simulink model "enginespeed_qat_mlfcn"  (R2025b)
settings: Solver=ode23  StartTime=0.0  StopTime=25  FixedStep=0.1  MaxStep=0.01  RelTol=1e-3  EnableMultiTasking=on
model workspace (MAT data in the model file):
  p = [-7.82997288351e-05; 0.181210895977; -0.072497134344; 0.000486358314052; 0.0361674637937]
settings Model: Creator=The MathWorks, Inc.  LastModifiedBy=arkadiyturevskiy
settings SolverCC: ZeroCrossAlgorithm=Non-adaptive  AlgebraicLoopSolver=TrustRegion
settings DataIOCC: LimitDataPoints=on  SaveFormat=Array  SaveOutput=off  SaveTime=off  ReturnWorkspaceOutputs=off
settings OptimizationCC: DefaultParameterBehavior=Inlined  InlineInvariantSignals=on  BufferReuse=off  ReuseModelBlockBuffer=off  ExpressionDepthLimit=2147483647.0  InitFltsAndDblsToZero=on  EfficientMapNaN2IntZero=off  LifeSpan=inf
settings DebuggingCC: SaveWithParameterizedLinksMsg=none  UnderspecifiedInitializationDetection=Classic  MergeDetectMultiDrivingBlocksExec=none  CheckExecutionContextPreStartOutputMsg=on  SignalResolutionControl=TryResolveAllWithWarning  MultiTaskDSMMsg=warning  FcnCallInpInsideContextMsg=warning  UnconnectedInputMsg=warning  UnconnectedOutputMsg=warning  UnconnectedLineMsg=warning  StateNameClashWarn=warning  SubsystemReferenceDiagnosticForUnitTest=warning  SFUnexpectedBacktrackingDiag=warning  SFNoUnconditionalDefaultTransitionDiag=warning  SFExecutionAtInitializationDiag=none  ArithmeticOperatorsInVariantConditions=warning
settings HardwareCC: ProdBitPerPointer=32.0  ProdBitPerSizeT=32.0  ProdBitPerPtrDiffT=32.0  ProdLargestAtomicFloat=None  ProdIntDivRoundTo=Undefined  ProdEndianess=Unspecified  ProdWordSize=32.0  ProdHWDeviceType=32-bit Generic
settings ModelReferenceCC: PropagateSignalLabelsOutOfModel=off
settings SFSimCC: SimParseCustomCode=off  CustomCodeUndefinedFunction=UseInterfaceOnly
settings RTWCC: GPUComputeCapability=3.5
settings CodeAppCC: StateflowObjectComments=on
settings GRTTargetCC: TargetFcnLib=ansi_tfl_tmw.mat  TargetLangStandard=C89/C90 (ANSI)  CombineOutputUpdateFcns=off  GRTInterface=on
settings ConfigComp: CovMetricSettings=dw  CovSaveCumulativeToWorkspaceVar=on  CovSaveSingleToWorkspaceVar=on

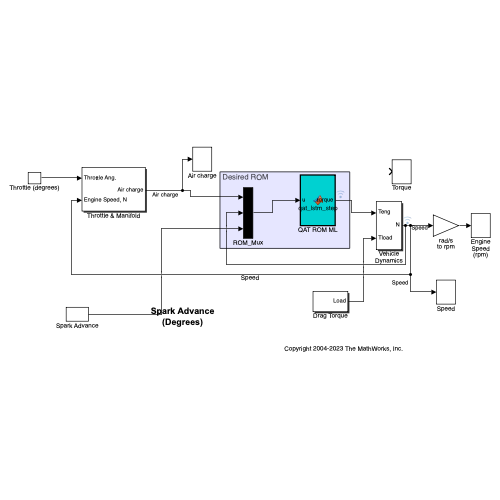
[thumbnail: Simulink's stored preview of the top-level diagram]
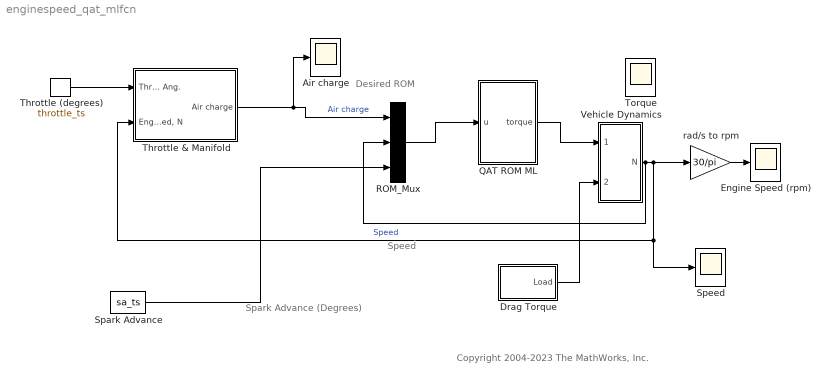
== system enginespeed_qat_mlfcn ==
  note: Speed
  note: Desired ROM
  note: Spark Advance
      | (Degrees)
  note: Copyright 2004-2023 The MathWorks, Inc.
  Air charge : Scope
      settings: ActiveDisplayYMinimum=0.13331  ActiveDisplayYMaximum=0.16893  DataLoggingVariableName=AirCharge  DataLoggingSaveFormat=Structure
  Drag Torque : Subsystem
  Engine Speed (rpm) : Scope
      settings: ActiveDisplayYMinimum=1212.0540686349664  ActiveDisplayYMaximum=9095.3798696194463  DataLoggingVariableName=N  DataLoggingSaveFormat=Structure
  QAT ROM ML : MATLAB Function  TreatAsAtomicUnit=on
  ROM_Mux : Mux  Inputs=3
  Spark Advance : FromWorkspace  VariableName=sa_ts  OutDataTypeStr=double  Interpolate=off  OutputAfterFinalValue=Holding final value
  Speed : Scope
      settings: ActiveDisplayYMinimum=198.02615  ActiveDisplayYMaximum=255.46189  DataLoggingVariableName=Speed  DataLoggingSaveFormat=Structure
  Throttle & Manifold : Subsystem
  Throttle (degrees) : FromWorkspace  VariableName=throttle_ts  OutDataTypeStr=double  Interpolate=off  OutputAfterFinalValue=Holding final value
  Torque : Scope
      settings: ActiveDisplayYMinimum=16.84896  ActiveDisplayYMaximum=31.50566  DataLoggingVariableName=Torque  DataLoggingSaveFormat=Structure
  Vehicle Dynamics : Subsystem
  rad/s to rpm : Gain  Gain=30/pi  SaturateOnIntegerOverflow=on  OutDataTypeStr=Inherit: Same as input  ParamDataTypeStr=Inherit: Same as input
  wires:
  rad/s to rpm/1 -> Engine Speed (rpm)/1
  Drag Torque/1(Load) -> Vehicle Dynamics/2(Tload)
  Throttle & Manifold/1(Air charge) -> Air charge/1, ROM_Mux/1  "Air charge"
  Vehicle Dynamics/1(N) -> rad/s to rpm/1, Speed/1, Throttle & Manifold/2("Engine Speed, N"), ROM_Mux/2  "Speed"
  Throttle (degrees)/1 -> Throttle & Manifold/1(Throttle Ang.)
  Spark Advance/1 -> ROM_Mux/3
  ROM_Mux/1 -> QAT ROM ML/1(u)
  QAT ROM ML/1(torque) -> Vehicle Dynamics/1(Teng)

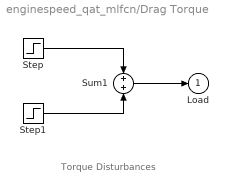
== system enginespeed_qat_mlfcn/Drag Torque ==
  note: Torque Disturbances
  Step : Step  Time=2  Before=25  After=25  SampleTime=0
  Step1 : Step  Time=8  After=0  SampleTime=0
  Sum1 : Sum  InputSameDT=on  SaturateOnIntegerOverflow=on  OutDataTypeStr=Inherit: Same as first input
  Load : Outport  InitialOutput=0
  wires:
  Step1/1 -> Sum1/2
  Step/1 -> Sum1/1
  Sum1/1 -> Load/1

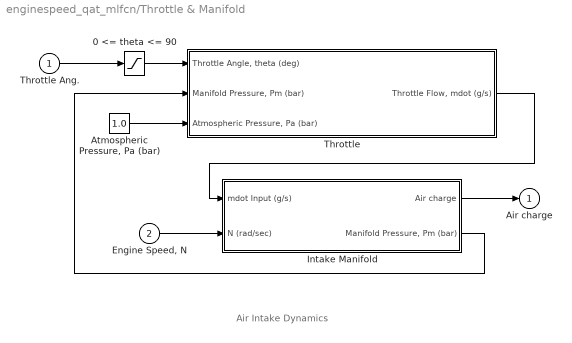
== system enginespeed_qat_mlfcn/Throttle & Manifold ==
  note: Air Intake Dynamics
  Throttle Ang. : Inport
  "Engine Speed, N" : Inport  Port=2
  0 <= theta <= 90 : Saturate  UpperLimit=90  LowerLimit=0
  "Atmospheric Pressure, Pa (bar)" : Constant  Value=1.0
  Intake Manifold : Subsystem
  Throttle : Subsystem
  Air charge : Outport  InitialOutput=0
  wires:
  "Atmospheric Pressure, Pa (bar)"/1 -> Throttle/3("Atmospheric Pressure, Pa (bar) ")
  Intake Manifold/1(Air charge) -> Air charge/1
  Intake Manifold/2("Manifold Pressure, Pm (bar)") -> Throttle/2("Manifold Pressure, Pm (bar)")
  "Engine Speed, N"/1 -> Intake Manifold/2(N (rad/sec))
  Throttle/1("Throttle Flow, mdot (g/s)") -> Intake Manifold/1(mdot Input (g/s))
  Throttle Ang./1 -> 0 <= theta <= 90/1
  0 <= theta <= 90/1 -> Throttle/1("Throttle Angle, theta (deg)")

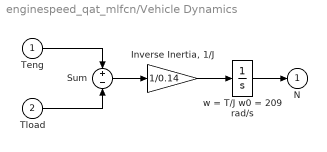
== system enginespeed_qat_mlfcn/Vehicle Dynamics ==
  Teng : Inport
  Tload : Inport  Port=2
  "Inverse Inertia, 1/J" : Gain  Gain=1/0.14  SaturateOnIntegerOverflow=on  OutDataTypeStr=Inherit: Same as input  ParamDataTypeStr=Inherit: Same as input
  Sum : Sum  Inputs=+-  InputSameDT=on  SaturateOnIntegerOverflow=on  OutDataTypeStr=Inherit: Same as first input
  w = T/J w0 = 209 rad/s : Integrator  InitialCondition=209.48
  N : Outport  InitialOutput=0
  wires:
  "Inverse Inertia, 1/J"/1 -> w = T/J w0 = 209 rad/s/1
  w = T/J w0 = 209 rad/s/1 -> N/1
  Sum/1 -> "Inverse Inertia, 1/J"/1
  Teng/1 -> Sum/1
  Tload/1 -> Sum/2

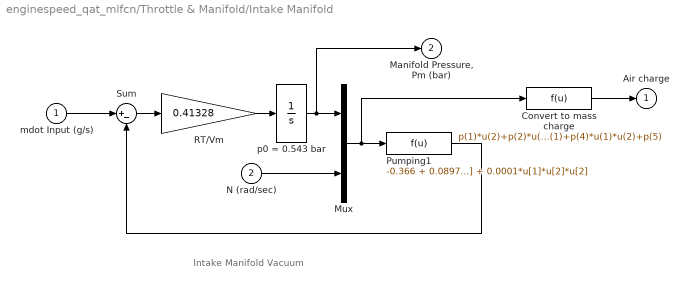
== system enginespeed_qat_mlfcn/Throttle & Manifold/Intake Manifold ==
  note: Intake Manifold Vacuum
  mdot Input (g/s) : Inport
  N (rad/sec) : Inport  Port=2
  Convert to mass charge : Fcn  Expr=p(1)*u(2)+p(2)*u(1)+p(3)*u(1)*u(1)+p(4)*u(1)*u(2)+p(5)
  Mux : Mux  Inputs=2
  Pumping1 : Fcn  Expr=-0.366 + 0.08979*u[1]*u[2] - 0.0337*u[2]*u[1]*u[1] + 0.0001*u[1]*u[2]*u[2]
  RT/Vm : Gain  Gain=0.41328  SaturateOnIntegerOverflow=on  OutDataTypeStr=Inherit: Same as input  ParamDataTypeStr=Inherit: Same as input
  Sum : Sum  Inputs=|+-  InputSameDT=on  SaturateOnIntegerOverflow=on  OutDataTypeStr=Inherit: Same as first input
  p0 = 0.543 bar : Integrator  InitialCondition=.543
  Air charge : Outport  InitialOutput=0
  "Manifold Pressure, Pm (bar)" : Outport  Port=2  InitialOutput=0
  wires:
  Pumping1/1 -> Sum/2
  Sum/1 -> RT/Vm/1
  p0 = 0.543 bar/1 -> "Manifold Pressure, Pm (bar)"/1, Mux/1
  Mux/1 -> Pumping1/1, Convert to mass charge/1
  N (rad/sec)/1 -> Mux/2
  RT/Vm/1 -> p0 = 0.543 bar/1
  mdot Input (g/s)/1 -> Sum/1
  Convert to mass charge/1 -> Air charge/1

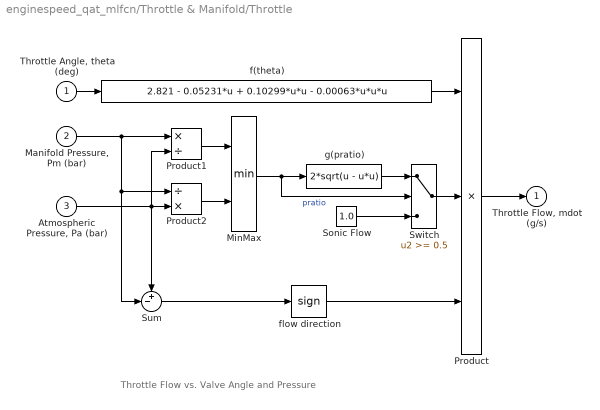
== system enginespeed_qat_mlfcn/Throttle & Manifold/Throttle ==
  note: Throttle Flow vs. Valve Angle and Pressure
  "Throttle Angle, theta (deg)" : Inport
  "Manifold Pressure, Pm (bar)" : Inport  Port=2
  "Atmospheric Pressure, Pa (bar) " : Inport  Port=3
  MinMax : MinMax  Inputs=2  InputSameDT=on  SaturateOnIntegerOverflow=on
  Product : Product  Inputs=3  InputSameDT=on  RndMeth=Zero  SaturateOnIntegerOverflow=on  OutDataTypeStr=Inherit: Same as first input
  Product1 : Product  Inputs=*/  InputSameDT=on  RndMeth=Zero  SaturateOnIntegerOverflow=on  OutDataTypeStr=Inherit: Same as first input
  Product2 : Product  Inputs=/*  InputSameDT=on  RndMeth=Zero  SaturateOnIntegerOverflow=on  OutDataTypeStr=Inherit: Same as first input
  "Sonic Flow " : Constant  Value=1.0
  Sum : Sum  Inputs=+-|  InputSameDT=on  SaturateOnIntegerOverflow=on  OutDataTypeStr=Inherit: Same as first input
  Switch : Switch  Threshold=0.5
  f(theta) : Fcn  Expr=2.821 - 0.05231*u + 0.10299*u*u - 0.00063*u*u*u
  flow direction : Signum
  g(pratio) : Fcn  Expr=2*sqrt(u - u*u)
  "Throttle Flow, mdot (g/s)" : Outport  InitialOutput=0
  wires:
  f(theta)/1 -> Product/1
  Product/1 -> "Throttle Flow, mdot (g/s)"/1
  "Throttle Angle, theta (deg)"/1 -> f(theta)/1
  MinMax/1 -> g(pratio)/1, Switch/2  "pratio"
  Sum/1 -> flow direction/1
  flow direction/1 -> Product/3
  Switch/1 -> Product/2
  "Sonic Flow "/1 -> Switch/3
  g(pratio)/1 -> Switch/1
  "Atmospheric Pressure, Pa (bar) "/1 -> Product2/2, Sum/1, Product1/2
  Product1/1 -> MinMax/1
  Product2/1 -> MinMax/2
  "Manifold Pressure, Pm (bar)"/1 -> Product1/1, Product2/1, Sum/2

== matlab function enginespeed_qat_mlfcn/QAT ROM ML ==
  data: u input; torque output
function torque = qat_lstm_step(u)
%#codegen
% QAT LSTM-32 ROM - Engine Torque from [AirCharge, Speed, SparkAdv]
% Platform-independent: no MEX compilation required.
% u(1) = AirCharge [g/s], u(2) = Speed [rad/s], u(3) = SparkAdvance [deg]
persistent h c
if isempty(h)
    h = zeros(32,1);
    c = zeros(32,1);
end

x = [(u(1)-0.21671053)/0.12929910; ...
     (u(2)-580.25021710)/235.62429395; ...
     (u(3)-15.0)/7.07177361];

S_WIH = 0.00476792; S_WHH = 0.00412825; S_WFC = 0.00407627;
BFC   = single(0.06805998);

WIH_raw = int8([62, 60, 11, -7, 25, -3, 35, 35, 4, -45, 88, 12, 79, 97, 36, -51, 38, 13, 5, -5, 5, -46, 12, 41, -102, 92, -5, -53, 13, 9, 37, 5, 24, -37, 44, 5, -32, 17, -1, -52, 19, 7, -8, 58, 10, -21, 79, 22, -4, 25, -37, -43, 3, 10, -83, 76, -4, 33, 28, -23, -45, 8, 9, 35, -5, -21, -57, 12, -17, 8, 95, 14, 75, -71, -30, 6, -10, 30, 47, 98, -14, -8, 61, -30, 75, -37, 62, -72, -19, 23, -45, 53, 22, 48, 30, 13, 70, -19, 7, -57, -7, 8, 36, -32, -2, -57, -5, -11, 18, -4, 22, -4, -13, -26, 12, -47, 21, -61, -13, -7, -31, 6, 8, -34, -21, 23, 30, -27, 12, -15, 48, 13, -55, -7, -35, -40, -36, -38, -17, 23, 19, -35, 46, 1, 3, 32, -13, 17, 43, -24, -23, 26, -6, 1, 28, -12, -12, 26, 0, 3, 23, 5, -12, -27, 10, 16, 1, 19, 36, -17, -20, 48, 14, -14, -10, 14, -25, 12, 45, -38, 44, 11, 25, -10, 3, 22, -12, 11, -7, 36, -33, -5, 83, -16, 16, -56, 20, -7, 127, -37, 16, -48, 54, -1, 35, -88, 2, -80, 11, -8, 102, 10, -19, -62, 25, 5, -59, 53, -9, -52, -1, 30, -55, 16, -16, -34, 58, 1, -65, -10, -21, 66, -3, 17, 55, -23, 12, 1, -61, -15, 54, -43, 4, -49, 19, -12, 11, -30, 10, -1, -17, -4, -44, 13, -11, -10, 5, -17, -82, 26, 6, -50, 51, 3, 64, 53, -8, -47, 30, -28, 40, -58, 14, 2, 63, -15, 5, -24, 41, -79, 6, -4, -61, 40, -16, -102, 45, -3, 62, 23, 15, -56, -2, -14, 58, 16, -5, -39, 37, 5, 63, 95, 3, -74, -3, 24, 13, -3, 7, -30, 64, 35, -124, 99, 2, -24, 40, 65, 44, 41, -17, -63, 79, 10, -60, -33, -29, -81, -13, 4, -14, 40, -8, -61, 57, 7, -36, 63, -23, -41, 24, -15, -112, 30, -47, 25, 41, 4, -78, 30, 5, 86, 19, 13, -121, 12, 1, 16, 36, 42, 35, -33, -45, 59, 59, 11, 34, 28, -23, 0, 72, -5, 37, 3, 5, -49, 14, 27, -34, 50, 25, 21, 42, 33]);
WIH = double(reshape(WIH_raw, 3, 128)')';  % 128x3

BIH = [0.29167804, 0.12725484, 0.88883609, 0.31790090, 0.20949835, 0.32797366, 0.60922438, 0.09490706, 0.31271005, 0.29229388, 0.20611192, 0.20403458, 0.16589172, 0.25161567, 0.31780127, -0.09208871, 0.12665981, -0.00661702, 0.11788771, 0.14943697, 0.04940436, -0.01206084, 0.42691094, 0.09601384, 0.14094143, 0.18544723, 0.08014344, 0.00143105, -0.05432267, 0.27028424, 0.36936006, 0.69753474, 0.03516542, 0.12005550, -0.19412988, -0.11750918, -0.06189374, -0.15380409, -0.11573982, 0.12027437, -0.05884297, -0.08844370, -0.12313346, -0.06570386, -0.00100128, -0.07784322, 0.02001838, 0.04074968, 0.00713495, 0.08415944, 0.03606167, 0.13949245, 0.03793926, 0.15232068, 0.22357759, 0.11216389, 0.15764646, -0.06942623, -0.07960395, 0.04245948, 0.10259989, 0.15876454, -0.10091246, -0.24197185, 0.22527131, 0.06279900, 0.23243006, -0.06028172, 0.09200291, 0.00935348, 0.19605409, -0.14657739, 0.30965030, 0.14182743, -0.04664635, 0.21879293, -0.01160003, -0.13498566, -0.08934867, -0.14389126, -0.23149504, 0.17198549, -0.24663855, -0.21485224, 0.26143301, 0.25563926, 0.23745435, -0.11224543, 0.23867871, -0.19211723, 0.18468942, -0.12143966, 0.30354387, -0.05351415, 0.06620202, -0.09468297, 0.24122736, 0.19066939, 0.42039448, 0.10199735, 0.21656252, 0.32056025, 0.66175717, 0.21913747, 0.48750350, 0.08492506, 0.12556908, 0.11773076, 0.17173931, 0.25194708, 0.36998215, 0.04848684, 0.03366598, 0.06815151, 0.07936064, -0.12722892, 0.23527583, 0.12203429, 0.24355148, 0.14841120, 0.18378572, 0.12308410, 0.14154433, 0.16662994, 0.08230788, 0.22511950, 0.30878866, 0.42226502]';

BHH = [0.33197251, 0.15704812, 0.81195515, 0.04355484, 0.24300784, 0.42988005, 0.65459627, 0.24522306, 0.34017837, 0.05615406, 0.16690490, 0.07055378, 0.37352693, 0.09706128, 0.30745202, -0.01832379, 0.12979737, 0.27995554, 0.23693827, 0.03899089, 0.09513167, -0.04901680, 0.35978654, 0.29616460, 0.14634728, 0.16586739, -0.01875892, 0.08425456, 0.25787374, 0.32291704, 0.31941339, 0.83596015, -0.00541261, 0.11395301, 0.00115809, -0.10114168, 0.10573789, 0.03869330, -0.13451317, 0.14324152, 0.17164624, 0.15689008, 0.01652173, -0.07098768, -0.08908617, 0.08816599, -0.01551705, 0.11856510, 0.17480265, 0.02629547, -0.13827856, 0.04314731, 0.19797699, -0.03786768, 0.01008944, -0.01221977, 0.08539730, -0.08183050, 0.12968449, 0.04252712, -0.01728092, -0.05926171, -0.15783741, -0.08016565, 0.20913637, 0.10704622, 0.06271764, 0.07323278, 0.31870967, 0.05725355, 0.01536318, 0.07521663, 0.28954452, 0.00777754, -0.19680467, 0.09190771, 0.05701484, -0.13078281, 0.14331143, 0.11639345, -0.24621609, 0.13644737, -0.41364101, -0.13830054, 0.18518278, 0.20315397, 0.22538413, -0.09509233, 0.28443125, -0.15073763, 0.08926047, -0.00858567, 0.34752741, 0.02784781, 0.05806050, 0.09664929, 0.38550791, 0.23860367, 0.57902074, 0.35842705, 0.20873210, 0.23231427, 0.66441500, 0.31338546, 0.17773914, 0.22918013, 0.04455853, 0.03923322, 0.27038547, 0.28805679, 0.17403774, 0.13441631, 0.33743805, 0.25465587, -0.04282241, -0.03289827, 0.19334051, 0.11179481, 0.13127369, 0.18829188, 0.28742275, 0.11362782, 0.05579545, 0.18546784, 0.16352095, 0.31996110, 0.26853830, 0.40363374]';

WFC_raw = int8([83, -74, 87, -86, 110, -79, 83, -82, -100, -84, -94, -50, -75, 87, 54, 58, 46, -38, 69, -12, -69, 27, -65, -58, 51, -76, 54, -37, 32, -51, -94, -127]);
WFC = double(WFC_raw(:));

WHH_raw = int8([32, 72, -6, 29, 57, 5, 25, 1, 87, 40, -17, 36, -2, -34, -21, -50, -71, 67, -62, -43, 53, 5, 18, -45, 19, -28, 11, 23, 77, 10, 69, -46, 25, 35, 8, -2, 16, -15, 12, 22, 51, 15, -23, -2, -5, -10, 0, -27, -47, 55, -58, -10, 12, 44, 29, 2, 25, -9, -7, 55, 78, -16, -14, 3, 51, -23, 14, -21, 0, -19, 27, 0, -2, 10, -21, 7, -14, 13, 17, -27, -13, 7, -31, -29, 27, 26, 61, 1, 62, -36, -9, 34, 13, -40, 11, -14, 51, -6, -2, 26, -3, -19, 46, 2, 28, 40, 6, 33, 12, -10, -19, -11, -3, 50, -11, -35, -1, 2, 26, 32, 57, -8, -32, -6, 11, -3, 9, -53, 40, 12, -1, 7, 46, 1, 52, 21, 52, 53, -23, 74, 34, -54, -21, -27, -37, 40, -48, -54, 37, 59, 64, -8, -6, -23, -17, 70, 5, 9, 36, -24, 74, 27, 54, 61, 71, 7, 24, 37, 33, 37, -39, 12, 40, -27, -19, 18, -11, 73, -45, -66, 9, 16, 11, -31, 3, -81, -12, -12, 18, 26, 46, -40, 11, 31, -1, 16, 44, -2, 17, 37, 55, 23, -38, 40, 25, -26, -10, 11, -64, 35, -67, -48, 46, 4, 71, -16, 5, -11, -20, 3, 26, -19, 25, -21, 64, 55, 53, 9, 18, 41, 38, 18, 36, -18, -41, 71, 7, -29, -56, -40, -33, 12, -41, -19, -7, 42, 15, -35, 50, -15, 8, 10, 3, -15, -3, -41, 80, -16, 101, 23, 18, -26, 78, -23, 5, -12, -40, 4, 29, -4, 13, 7, -24, 4, -1, -14, -7, 46, -13, 1, 53, -49, 24, 27, 65, -40, -30, -52, 77, 35, 4, 50, 18, -5, -15, 3, 44, 20, -46, 39, -7, 17, -48, -28, -55, 15, -7, 5, 28, 62, 45, 17, 64, -13, -20, 52, 63, -15, -16, -54, 43, 1, 48, 51, -8, 22, 32, 32, 63, -22, 9, 79, 35, -56, -52, -38, -51, 60, -32, -9, 23, 45, 50, -40, -4, -55, 16, 9, -1, 27, 51, -8, -2, -28, 37, 41, 33, -14, 40, 28, -19, -24, 1, -17, -25, 30, 7, 8, -21, 11, 32, -38, -7, 40, -17, 22, 1, -32, -7, -17, -16, 12, 2, -50, 26, 56, 55, 35, 15, -9, 39, -5, 3, 11, -28, 25, 25, -37, -10, 12, -49, 0, -13, -31, 8, 70, 18, 13, 62, -79, 26, -16, 25, -2, -10, -1, 43, 36, 4, 45, 16, -20, 42, 29, 57, -11, -44, 39, 30, -7, 1, -15, -3, 62, -32, -8, 46, 66, 14, -19, 28, -44, 18, -4, 63, -6, 32, -37, 7, -6, 0, 37, -7, 0, 42, -16, 14, -32, -33, -7, -3, -25, -9, -14, -6, 57, 4, -41, -19, 40, 4, 19, 57, -16, 26, 50, 36, -24, 37, -45, -29, 15, 25, -2, -24, -54, -15, 31, -15, -2, -11, -16, -11, 30, 43, -18, 33, -7, 45, 21, -2, 30, 4, 16, -50, 23, -20, 7, -25, -7, -2, 2, 23, -12, 13, -6, 43, -7, 69, -10, 2, 7, -51, 20, -15, -12, -24, 13, 19, 21, 24, -29, -6, 26, 10, -8, -8, -17, -29, 23, 51, -24, -9, 2, 8, -7, 49, -6, -15, -34, 18, -16, -12, 9, -4, -4, -24, -12, -16, -21, -42, 14, -29, -36, -27, 28, -9, -19, 45, 7, 14, -21, -9, -18, 26, -9, -7, 24, 12, 12, -7, 41, 33, 10, 36, -5, -2, 41, 23, -20, 14, -24, -40, 46, 20, -1, 29, 29, 32, 53, -16, -18, -31, 30, 39, 8, -9, -27, 7, -38, 33, -22, 24, -19, 13, -40, 29, -30, -46, 13, -23, -8, 3, -11, -18, -7, -18, -28, -26, -2, 27, -8, -13, -4, 39, 22, -23, -29, -11, -28, 70, 10, 56, -4, 20, -22, 53, -9, -4, -21, -20, 57, 30, -36, -13, -14, -54, 52, 0, -22, 3, 11, 35, 21, 43, -54, 26, 10, 15, -11, 34, -33, 6, -7, -10, -20, 17, 3, 42, 17, 19, 8, -34, 28, 28, 19, 11, 20, -7, 29, -45, 12, 3, 9, -7, -44, -6, -28, 10, -28, 12, 5, 26, 23, -3, -17, 34, 29, -17, 15, 39, 14, -5, 39, 13, 31, 1, -1, -31, 25, -35, 38, -4, -9, 18, 27, 3, -23, 1, 12, -15, 14, 12, 41, 13, -7, -2, -6, 20, 8, 38, -13, 34, 49, 32, 32, -41, 69, -1, -52, 7, -41, -33, 57, -50, -49, 29, 12, 30, -33, 23, -29, -14, -4, 36, 13, -5, 5, 24, -1, -21, 7, 53, 26, -29, 37, 6, 31, 28, 26, -3, -2, -5, 12, -38, -7, -44, 14, 12, -37, 68, 1, 37, 1, 49, -13, 13, 17, 38, -19, 32, 18, 25, 21, 29, 32, 11, 35, 79, -7, -50, 16, -4, -32, -31, -43, -56, 18, -60, 8, 22, -3, 54, -17, 63, -5, 45, 10, 50, 26, 24, 7, 49, 20, 33, 6, -29, 6, 28, -12, 13, -15, 22, 63, 9, -33, 8, -11, -11, 25, 8, -34, 7, 13, 20, 30, -3, -13, 12, 18, 38, 6, -10, -27, -27, 9, -8, -38, -24, -12, -6, 22, -28, 16, 16, -35, -5, 43, -21, -28, 37, 17, 9, 23, -19, -35, -14, 32, -22, 22, -43, 46, 15, 9, -34, 13, -12, -12, -12, -4, -7, 14, 25, -15, 42, 20, 17, 27, 22, -16, 20, 15, -33, -21, -38, 22, -5, -8, 27, -11, -8, 9, 38, -26, 6, -3, 32, 46, 38, 8, 58, 10, 25, 12, -2, 17, 2, 13, -26, 33, -12, -54, -9, 16, -59, 43, -44, -25, 58, 45, 6, -7, 50, -37, 46, 8, 22, -16, 21, -16, 28, -12, 24, 29, -19, -10, 24, -4, 15, 1, 5, 12, -16, 17, -9, -11, -44, 29, -17, -28, 29, 6, -12, -18, 59, 3, -10, 57, 21, -33, 10, -41, 64, 14, 54, 31, 63, -46, 51, -32, 44, -14, -54, 44, -11, -28, -18, -18, -5, 22, -13, -31, 13, 35, 12, -55, 26, -76, 2, 32, 22, -36, 1, -25, -15, 1, -6, -13, 7, -26, -12, -7, -38, 12, -8, 11, -3, 36, 15, -22, 23, -34, -12, 3, -9, -47, 42, 8, 18, 34, -20, -3, 26, 15, -1, 25, 0, 5, 11, -32, -45, -37, 39, 8, -56, -9, -9, -28, 10, 39, 7, -36, 6, 19, 60, -37, -34, 37, 1, -3, -7, -30, 22, 11, 41, 35, 1, -15, -2, -3, -42, -10, -17, -23, -2, -43, -67, 5, -28, -59, -37, 21, 47, 31, 30, -19, 48, 9, -54, -58, -62, -32, -47, 18, 17, 33, 3, -26, -17, -8, 34, -31, 31, 20, 2, 18, -6, 41, 2, 33, 9, 34, 25, 13, 20, -15, 20, 15, 41, 25, 12, -5, 1, 28, 16, -15, 14, 32, -18, 4, 3, -43, 11, -1, -14, -1, -15, 58, 15, 50, 14, 27, 19, 16, -15, -34, -18, -10, 10, 17, 7, 7, 2, -56, -20, -26, 26, 24, 44, -2, -2, -2, 42, 4, -5, 4, 15, 7, -22, -22, -3, -19, -66, 26, 11, -32, -17, -5, -31, 23, 20, 12, 52, 14, 2, 5, -35, 39, -5, -12, -1, -25, -25, -19, -52, 39, -38, 3, -40, -21, 6, 4, -21, 5, -8, 18, 4, -5, -22, -9, 34, -1, 23, -11, 39, 16, -37, -26, 11, 8, 26, -5, 23, -46, 9, 11, -2, -3, -10, 1, -23, -36, -46, -1, 9, 5, -41, 19, -10, -9, -26, -9, 38, -25, 21, -41, 39, -5, 1, -30, 8, -10, 18, -16, 15, -22, -11, -6, 17, -6, 34, 14, 45, 17, 32, -23, 37, -8, -14, 6, -27, 32, 3, -18, 21, -24, -22, 12, 20, -16, 12, 40, -21, -2, 2, -29, -8, 21, 50, 9, -32, -71, 10, 20, 12, -13, -44, 13, 18, -18, -7, 32, 19, -8, -9, 33, 26, 35, 1, 10, 73, -37, 7, -4, 22, 0, -4, 19, -51, -25, -14, 31, 14, -43, 13, -25, -17, 30, 16, 0, 10, 9, -15, -12, -20, 19, 14, 20, -6, 31, 34, 17, 26, 44, -7, -26, 32, 45, -11, 40, 17, -6, 31, -12, 60, 33, -1, -24, -20, 0, -19, -33, 34, 20, 2, 16, -9, -22, -41, 9, 35, 0, -6, -18, 5, -44, 18, 13, -31, -3, 15, -29, 14, 25, -12, -33, -7, -53, -50, 27, -1, -27, -16, -26, 27, -17, -39, -29, 24, -36, 5, -17, -17, 28, 45, -20, 36, -3, -18, 14, -11, 43, -13, 0, -23, 15, -36, 29, 14, 15, 19, -8, 37, -29, -29, 32, 7, -5, -27, -18, 18, -14, 5, 3, 29, -9, -5, 29, 56, -22, -37, 13, 23, 25, 29, -28, 9, -27, 28, 39, 16, 8, -1, -27, -15, 29, -6, -33, 32, 31, -55, 32, -2, 13, 23, 41, 11, 24, 14, 14, -5, -13, -27, 34, 4, 18, -21, -28, 14, 29, 27, -10, -8, -42, 38, -16, 34, 25, -55, -23, -4, -25, -14, 0, 15, -21, -12, -10, -3, -7, 36, 4, 8, -6, -40, 6, -38, 9, 29, -37, -46, 21, 5, -16, 11, -46, 8, -27, 19, -16, 23, -37, 46, -33, 14, 17, -59, 4, -58, 39, -20, -37, 31, -31, 41, -12, 20, -7, 24, 12, 22, 5, -44, -1, 45, -38, -25, -30, 1, -10, -15, 16, -21, -16, 42, 5, 9, 1, -18, -2, -17, -21, -21, 26, -13, 18, 23, -11, -21, -6, -8, 8, -22, -12, 8, 42, 23, 1, 27, 7, 25, 11, 12, 4, -9, 4, 16, 27, 39, -11, -38, 7, -13, 27, -28, -28, -32, -2, 28, -48, 6, 13, -3, 40, 14, -21, -13, 25, -1, -14, -13, -81, 42, -47, -17, -24, 21, -44, 39, -45, -15, -21, -57, -26, -28, 42, 63, 32, -7, -36, 15, -18, -45, -43, 2, 6, 2, -31, -8, -12, 5, -21, -4, 30, 27, 17, 22, 26, 5, -43, -10, 4, -4, 27, -28, -37, 1, -8, 5, -13, 18, 12, 52, -45, 22, 21, -15, 34, -24, 19, -15, 18, 33, 10, 17, -3, -5, 24, -1, 3, 53, 7, 15, -23, 63, -21, -19, 14, 18, 19, -20, -15, 6, 21, -59, -37, 42, 16, 23, -58, 9, -14, 28, 27, 15, -18, 14, -1, 8, 23, 47, 32, 35, 29, 19, 34, 29, 18, 28, 48, 35, -24, 8, -35, -1, 42, -4, -21, 1, 35, 7, 17, 42, -51, -5, -5, 50, -4, 33, 11, 25, 43, 11, -31, 23, 18, 2, -32, -40, -2, 48, 27, 30, 22, -26, -21, -15, -18, 40, 17, 35, -18, -39, -1, 34, 33, 11, -5, -43, -6, 35, -24, 26, 1, -15, 16, -1, -7, -18, -34, -18, 18, -18, 13, -38, -38, 0, -5, 3, -20, -3, -11, -3, -42, 24, 22, 33, -27, -11, -21, -22, 14, 39, 40, 24, -15, 6, -4, 1, 28, -27, 7, -28, -23, -11, 18, 25, 13, 19, -3, -8, -13, -5, 45, 15, -64, 6, -31, 4, -31, 24, -29, 33, 26, 7, -36, 7, -8, 19, -24, 6, -38, -21, -12, -7, 23, -38, -21, -24, -36, 10, 3, -4, -21, 5, -33, -23, -16, 36, 3, 26, -12, -19, -17, 33, 57, 31, 7, 41, 22, 34, -36, -60, -50, 18, -43, -69, -15, -40, 2, -16, 1, 35, -19, -16, 12, 68, -13, -43, -18, -5, 45, 23, -12, -50, -13, -16, -9, -49, -49, 18, -35, -34, -14, 2, 12, 19, 3, 25, 11, -11, -18, -15, -15, 4, -21, 0, -18, -6, 36, 14, -15, 7, -8, -16, -20, 9, -14, -32, 9, 36, -4, 4, -9, -5, -3, 28, 11, -36, -12, -10, 25, 5, -19, -13, -16, -17, 20, 27, 17, 17, 14, 21, -5, -3, 11, -7, -21, 16, -34, 23, 45, 9, 30, -17, 29, 41, 3, -31, -22, 11, -2, -48, 8, -13, -22, -19, -3, -41, -13, 4, 20, 62, -26, 10, -2, -42, 11, -32, -27, -44, -1, 21, 18, -35, -38, -48, -47, -48, -10, -1, -38, -4, -45, -90, -4, -11, -23, 7, 19, 0, 31, -3, -15, 39, 59, -73, -81, -27, 7, -2, 47, 5, -13, -35, -24, -26, -2, -25, 30, -41, 35, 21, 15, 36, -17, 42, 20, 9, -15, 15, -25, 2, 21, -8, -2, -70, 59, 41, -7, 10, -42, 54, 22, 48, -52, 30, -8, 102, 87, 12, -18, 57, -11, 35, -55, -2, -32, -13, 17, -46, -30, 39, 8, -10, -24, -23, 3, 34, -38, -1, 7, 1, 16, 39, -15, -16, 44, 35, -16, -22, -25, 22, 10, -53, -5, 47, -20, -51, -12, -12, -14, -57, -4, -5, -16, -5, 39, -18, 5, -13, 13, -8, -20, 72, -29, 24, -47, -8, 10, 7, 45, 42, 50, 28, 44, 13, -19, -10, -18, 25, 6, -5, 32, 19, -40, 45, 13, -35, 40, 7, -1, 0, -20, -35, 41, 35, -3, 34, -16, -6, -29, 8, 25, -6, -11, -15, 24, 15, -1, -5, 22, -16, 41, 50, 7, -1, 34, 11, 26, 30, -33, 4, -34, -91, 27, 22, -22, 72, -38, 3, -13, 22, -20, 40, -19, 51, 35, 40, 19, 40, 18, 30, 8, 47, -9, -70, -21, 22, 19, -1, 23, 9, 4, -11, 0, 89, -28, 22, -18, -24, 17, 26, 20, -9, -31, 21, -26, -59, -27, -29, 53, -48, 42, 31, 18, 1, 39, 62, 56, -4, -3, 55, -16, -41, 50, -48, 15, -27, 31, -2, -10, -2, -30, 47, -16, -1, -43, 13, 1, 31, 33, 7, -20, 25, -9, -38, -21, -24, -38, -46, -37, -31, 16, 5, -24, 5, 31, -40, -16, 19, -25, -5, -12, 12, -15, 31, -21, -22, 13, -10, 44, -66, -45, -2, 40, 105, 50, 11, -14, 65, 4, 42, 4, -34, -9, 53, -18, -36, -6, -48, 35, 3, -68, 45, 20, 48, -29, 38, 7, 25, 26, 86, 48, -13, -53, -3, 38, 42, -7, -13, -24, 15, -34, 6, -13, 18, 11, -19, 11, 11, -32, 37, 41, 52, -19, 15, -3, -13, 31, 15, 17, -51, 35, -8, 42, 8, -3, 31, 27, 20, -9, 26, 3, 19, -7, 20, 36, -31, 24, -34, -31, -42, 15, -30, -18, 12, -6, -46, 3, -17, 16, -39, 23, -40, -37, -2, -20, -9, -41, 29, 15, 5, 36, 1, -25, -3, -14, -23, -37, -11, 0, 40, 22, 32, 14, 12, 45, 41, -53, -5, -16, 19, -23, 64, -34, 4, -27, 2, 3, -21, -47, 32, -5, 17, 37, 7, -35, 19, 16, -52, 14, -2, 17, 26, -26, 18, -37, -51, 39, 12, -26, 28, -9, -31, 28, 43, -16, 17, 37, 33, -27, -11, -13, 11, 19, -58, 1, -9, 7, 13, 16, 20, -43, -24, -8, -3, -29, 50, 13, -17, 9, -9, 1, 15, -48, 7, 28, 26, 27, 5, -3, -3, 5, 21, 32, -13, -39, -52, -37, -17, 54, 2, -29, -1, 7, -8, -15, -9, -9, 8, 14, 44, 17, -4, 25, -21, -33, -15, 4, 7, -18, -20, 6, 10, 41, 27, 39, 4, -29, -38, 10, -18, 30, 9, 8, 35, 20, 19, 19, -21, -12, 1, 24, 33, 22, -25, 5, -33, 12, -38, -24, 26, 22, -9, -37, -39, 27, -31, 47, 20, 10, -39, 48, 21, 60, 30, -16, 26, 6, -16, 33, -14, -17, -15, 13, -10, -15, 15, 42, -11, -19, -23, -38, -40, -3, 39, -42, -18, -21, -41, -2, 27, -8, 60, 21, 41, -8, 27, 18, -24, 20, -7, -3, -12, -29, -31, -15, -5, -8, 6, -47, -21, 43, -18, -4, 54, 0, 13, -19, 32, -24, -14, 10, -13, -61, -72, 2, 19, 21, 9, -63, -7, 17, 11, -18, -52, -5, 53, -18, 42, -31, 12, 29, -59, -31, 13, -17, -2, -24, 52, -22, -34, -12, -25, 32, -38, 20, -33, 22, -84, 52, 4, 24, -23, -10, 51, 20, 45, -3, -2, 40, 9, -25, -5, 16, 25, 33, -50, 51, -46, 31, -5, -46, 11, 38, -32, 26, -3, 16, 25, -25, -15, 10, 10, -13, -14, 16, -15, -21, -19, -15, 7, 23, -24, 28, 47, -45, -7, 48, 41, 26, -16, 14, -54, 37, 32, 21, -47, -45, 43, 20, 9, 33, 30, -39, 8, -10, 37, 7, -52, 24, -47, 37, 1, -42, -14, 10, -19, -9, 32, -16, 40, -34, 44, -6, 22, 39, 52, -40, 21, -29, 44, 3, 49, 15, -3, -24, -23, -17, 36, 24, 20, -17, 18, -61, -6, 13, -62, 58, -50, 10, 28, 54, 64, -22, 17, -9, -26, 20, 9, 48, -13, -47, 23, -25, 33, 31, 32, -56, -2, -13, -15, -35, 19, -13, -27, -34, 22, -8, 33, -1, 56, -16, -18, -1, -42, 27, -39, 22, -24, 23, 41, -27, 11, -12, -23, 15, 32, 28, -39, 29, 24, 46, 24, -13, 28, 66, -41, -9, 33, 13, -10, 31, -37, -2, -10, -15, 30, -37, 2, -38, -24, 34, -27, 19, 19, -7, -10, 39, -1, 44, 6, 17, -35, -16, -58, -15, -2, -2, 32, 21, -39, -27, 30, 3, 57, -40, -12, 35, -48, 44, 8, -23, -38, 2, 8, -13, 0, -59, -9, -21, 23, 3, 0, 44, -25, 10, -6, -6, -46, -22, -32, 22, -13, 10, -23, -7, -29, 46, 0, 8, 20, 25, 44, 7, -14, -7, 15, 20, 29, 32, -35, 16, -5, -23, -20, -39, 6, -20, -28, 1, -24, -6, -7, 8, 22, -14, 29, -3, -3, -19, 6, 17, 3, -23, 19, 0, -39, -16, -8, -16, -41, -31, 61, -38, 48, -26, 17, -21, -6, 15, 52, -28, -38, 41, -10, 3, 26, -20, -39, 22, -46, -26, -9, -21, 78, -14, 45, -22, -4, 24, 13, -20, 51, -17, 5, -48, 38, 16, -40, 10, 7, -27, -5, 9, 10, -28, -26, -24, 25, 9, -21, 28, 70, -28, 7, -7, 12, 45, -41, -29, -20, 11, -20, -32, -27, -34, 15, 1, 36, 18, -24, -16, 38, 34, -54, -25, 23, -29, 21, 26, 4, -26, -6, -38, 10, 11, -43, -18, -33, 25, 1, -18, -32, 14, 42, 36, -16, -52, 39, 9, 81, -23, 4, -41, 39, -33, 14, 23, 39, -18, 32, -23, -29, -12, -44, -12, -5, -56, 36, 80, 3, 33, -36, -24, 8, 28, 3, -22, -60, -78, 19, 46, 26, 43, 27, -8, 46, 29, 79, -8, -63, 45, 11, -16, 16, -25, -80, 35, -41, -24, 35, 30, 13, -44, 65, -54, 47, 3, 73, 8, 79, -18, 36, 3, 11, -4, 33, -10, 27, -24, 27, 4, -41, 35, -27, -21, -49, 1, -58, 35, 3, -63, 48, 66, 7, 13, 43, 3, 17, -7, 5, -28, -11, -35, 9, 15, -9, -24, -13, -66, 58, -12, -19, -35, -61, 16, -15, 54, 42, -22, -45, -2, 11, -59, 1, 15, 58, 6, 21, -62, 6, 9, 19, -20, 28, -39, 17, -13, -6, 31, -6, 11, 19, -11, 36, 35, 14, 70, -21, -37, -53, 3, -5, 60, -33, -54, 59, 2, 1, 30, -2, -45, -2, 60, 28, -26, 34, 6, -3, 38, -8, 33, 30, 42, 52, -11, 46, 38, -21, 42, -6, 13, -74, -66, -18, 14, -45, -54, 39, 7, 70, 12, 38, -23, 4, 24, 10, 10, 47, -3, 45, 30, 10, 50, 14, 31, 50, 32, 68, 32, -42, 12, -6, -16, -18, -53, -30, 28, -22, -54, 68, 67, 67, 21, 52, -40, -32, 23, 39, 34, 15, -18, 44, 21, 32, 19, 41, 0, 39, 8, 42, -6, 9, 31, 34, -44, -33, -9, -60, 36, -48, -31, 58, 34, 16, -48, 46, -48, 20, 2, 37, -11, 29, -24, 12, 4, 37, 53, 33, 16, 48, 48, 13, -16, -15, 43, -16, -57, -23, 14, -63, 12, -29, -66, 2, 51, 62, -26, 33, -68, 15, 4, 14, -8, 25, -10, 88, 18, 127, -8, 29, -24, 104, -15, -4, -38, -40, 33, -10, 35, 14, 1, -35, 40, 67, -72, -33, 30, -21, 14, 41, -63, 32, 49, 28, -68, -57, -112, 32, 26, 7, 35, 17, 43, 30, -13, -18, 7, -31, 38, -12, -51, -8, 7, -32, -15, 6, -9, 53, 25, 57, -20, 65, -53, -46, 47, 24, 40, -14, -1, 67, 33, 56, 6, 16, 18, 56, -5, 53, -4, -43, 44, -12, -56, -16, -7, -20, 25, -60, -62, 65, -12, 43, 14, 65, -55, 3, 9, 52, -41, 6, -58, 57, 14, 51, 35, -5, -45, 12, 3, 7, -4, -49, 10, -32, 9, -4, -4, -37, 37, 7, -12, 12, 41, 24, 15, 45, -22, 19, -3, 0, 2, -11, -25, 13, 35, 63, 14, 41, 27, 5, -3, 8, -11, -5, 64, 27, 4, -48, 5, -31, 11, -12, -27, 23, 49, 49, 31, 39, -43, -2, 28, 18, 3, -15, -65, 14, 50, 17, 17, 21, 45, 45, -15, 51, -24, -13, 62, 51, -29, -45, 12, 9, 10, -9, -58, 38, 39, 49, -4, -4, -52, -42, 10, 53, -22, 8, -79, 17, -3, 21, 5, 25, 28, 59, 20, 14, 3, 3, 13, 33, -49, -49, -10, -48, 40, 16, -21, 58, 23, 10, 2, 28, -56, -11, 60, 17, 25, 24, -14, 4, -11, 20, -7, -48, 19, 26, -12, 26, 21, 9, 47, -30, 8, 17, -34, -10, -20, 57, 2, -15, 15, -8, 1, 4, -22, -27, 14, -20, 37, -14, 8, 30, 14, 50, 28, 27, -45, 26, 3, 25, 4, -24, 52, 15, 23, 12, -15, -43, 28, 4, -59, -6, 14, 3, 20, 67, -53, 7, 21, 45, -29, -25, -50, 72, 2, 5, 9, -16, -33, 70, -5, 15, -47, -34, 32, -34, -10, 23, 0, 5, -19, 24, -28, 6, 60, -22, -2, -13, 0, 11, 24, 12, -2, -25, -13, 54, 7, 54, 25, -9, 24, 70, -4, 37, 17, -10, 56, 42, 12, -22, 0, -54, 44, 5, -21, -9, 60, -20, 69, 36, -39, -31, 62, 43, 39, -11, -59, 41, -51, 35, -18, 53, -30, 16, 6, -24, -11, -18, -8, -22, -10, 2, 19, 20, -40, 5, 3, 18, -38, 2, -64, -16, -26, -7, 42, -7, -12, -46, -4, 13, 46, 80, 44, 1, 25, 2, 20, -15, -21, -41, -22, 21, -29, -27, 30, -30, 31, 19, -10, 25, 47, 29, 2, 63, -36, -34, 24, 32, -22, -3, -43, -8, -19, -18, -33, 43, -1, -12, -29, 6, -15, -37, -18, -9, -15, 42, 5, -6, -6, -22, 27, -23, -6, 34, -47, -23, -31, 33, -5, -20, -40, 5, 29, 45, 4, 36, -20, 15, 42, 22, -3, 29, -11, 2, -7, -20, -34, -23, -3, -17, 29, 6, 12, 20, 32, 36, 1, -20, 21, 12, -15, 11, 9, 36, 16, 52, 47, 19, 71, -6, 28, 14, -7, 7, 32, -14, 10, 5, -14, -60, -4, -67, 27, -66, -62, 23, 57, 65, 18, 58, -39, 15, 54, -17, -16, 40, -25, -3, -22, 45, 8, 29, -48, 53, -34, 22, -3, -18, 35, -1, -29, 46, -30, -6, 7, -70, 18, 36, -36, 74, -49, 62, -39, 66, 15, 24, 6, 49, -28, 44, 36, 13, 57, 18, -9, 0, 29, 24, 29, -53, 39, -18, 4, 7, -14, -41, -17, -58, -35, 56, -18, 45, 16, 43, -51, 14, 18, 37, -8, 44, 12, 34, 43, 9, 54, 17, -7, 34, -22, 16, 37, -54, 14, 25, -12, -20, -21, -45, 54, -41, -41, 47, -8, 16, 3, 13, 1, -35, 21, 5, 35, 40, -61, 16, 10, 42, 23, -35, 7, 9, -20, 3, 20, 11, -29, -26, 49, -15, -35, -41, -17, -9, -2, 12, 49, 17, 15, 24, 25, -46, 48, -29, 19, -44, -1, 29, 6, 14, -2, 40, -4, 6, -14, 27, -19, -30, 39, -4, -9, 14, -12, -43, 8, -76, -19, -10, 9, 15, -15, 55, -50, 5, -12, 28, -4, 25, 17, 48, -14, 27, 6, 34, 29, 27, -17, 42, -26, -45, 43, 48, 17, -30, -1, -61, 24, -30, -22, -1, 39, 52, 4, 25, -9, -18, 18, 49, 9, 27, -57, 52, -15, 29, 20, -26, -36, 10, 40, 22, -12, -21, -4, -27, -35, -56, 10, -44, 25, -22, -47, 14, 25, 40, 45, 15, -8, -27, 39, 56, -4, 28, -47, -3, -5, -21, 31, 11, -56, -3, -50, -28, 9, -3, 64, -26, -9, -16, -13, -53, 30, -60, -13, 45, 27, 65, -70, 23, -61, 21, 5, 6, -64, -7, -14]);
WHH = double(reshape(WHH_raw, 32, 128)')';  % 128x32

g = BIH + BHH + S_WIH*WIH*x + S_WHH*WHH*h;
ig = 1./(1+exp(-g(1:32)));
fg = 1./(1+exp(-g(33:64)));
gg = tanh(g(65:96));
og = 1./(1+exp(-g(97:128)));
c  = fg.*c + ig.*gg;
h  = og.*tanh(c);
torque = (double(BFC) + S_WFC*(WFC'*h)) * 46.99854266 + 25.94591248;
